simulink model "lab5_sim"  (R2024b)
settings: Solver=VariableStepAuto  StartTime=0.0  StopTime=0.3  RelTol=1e-3
values from neighbouring files (symbols this model uses):
  A = [-Ra/La, -K/La; K/J, 0;]    [Lab5.m]    (also in Lab5_recapitulare.m)
  A_d = double(expm(A_aux))    [Lab5.m]    (also in Lab5_recapitulare.m = double(expm(A * h)))
  B = [1/La, 0; 0, -1/J]    [Lab5.m]    (also in Lab5_recapitulare.m)
  B_d = double(int(expm(A * t) * B, 0, h))    [Lab5.m]    (also in Lab5_recapitulare.m)
  C = [1, 0; 0, 1]    [Lab5.m]    (also in Lab5_recapitulare.m)
  C_d = C    [Lab5.m]    (also in Lab5_recapitulare.m)
  D = [0, 0; 0, 0]    [Lab5.m]    (also in Lab5_recapitulare.m)
  D_d = D    [Lab5.m]    (also in Lab5_recapitulare.m)
  h = 0.01    [Lab5.m]    (also in Lab5_recapitulare.m)
undefined symbols (not defined in the file or in its folder): denz1, denz2, numz1, numz2
settings Model: Creator=akopo  LastModifiedBy=akopo

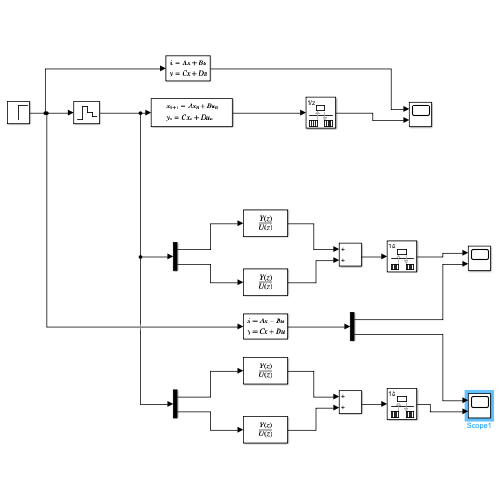
[thumbnail: Simulink's stored preview of the top-level diagram]
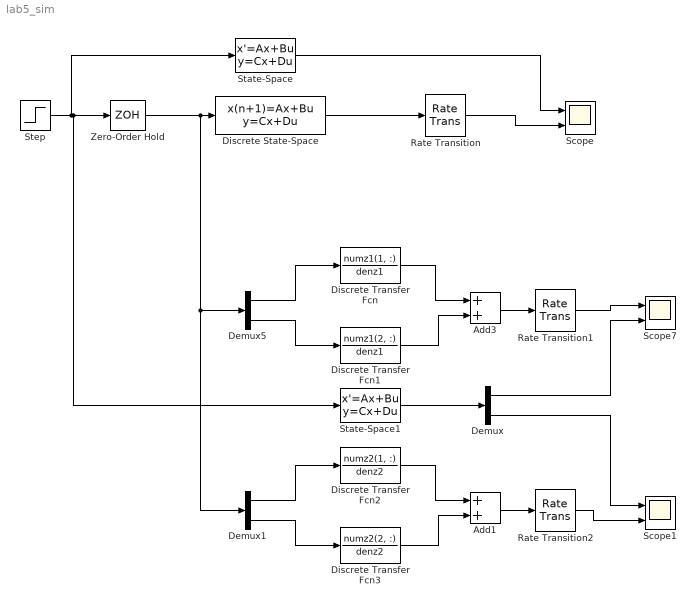
== system lab5_sim ==
  Add1 : Sum
  Add3 : Sum
  Demux : Demux  Outputs=2
  Demux1 : Demux  Outputs=2
  Demux5 : Demux  Outputs=2
  Discrete Transfer Fcn : DiscreteTransferFcn  Numerator=numz1(1, :)  Denominator=denz1
  Discrete Transfer Fcn1 : DiscreteTransferFcn  Numerator=numz1(2, :)  Denominator=denz1
  Discrete Transfer Fcn2 : DiscreteTransferFcn  Numerator=numz2(1, :)  Denominator=denz2
  Discrete Transfer Fcn3 : DiscreteTransferFcn  Numerator=numz2(2, :)  Denominator=denz2
  Discrete State-Space : DiscreteStateSpace  A=A_d  B=B_d  C=C_d  D=D_d  SampleTime=h
  Rate Transition : RateTransition
  Rate Transition1 : RateTransition
  Rate Transition2 : RateTransition
  Scope : Scope  NumInputPorts=2
  Scope1 : Scope  NumInputPorts=2
  Scope7 : Scope  NumInputPorts=2
  State-Space : StateSpace  A=A  B=B  C=C  D=D  InitialCondition=0
  State-Space1 : StateSpace  A=A  B=B  C=C  D=D  InitialCondition=0
  Step : Step  Time=0  Before=[0, 0]  After=[24; 0.04]  SampleTime=h
  Zero-Order Hold : ZeroOrderHold  SampleTime=h
  wires:
  Rate Transition/1 -> Scope/2
  Step/1 -> State-Space/1, State-Space1/1, Zero-Order Hold/1
  Discrete State-Space/1 -> Rate Transition/1
  State-Space/1 -> Scope/1
  Demux5/1 -> Discrete Transfer Fcn/1
  Demux5/2 -> Discrete Transfer Fcn1/1
  Discrete Transfer Fcn1/1 -> Add3/2
  Discrete Transfer Fcn/1 -> Add3/1
  Add3/1 -> Rate Transition1/1
  Rate Transition1/1 -> Scope7/1
  Rate Transition2/1 -> Scope1/2
  Demux1/2 -> Discrete Transfer Fcn3/1
  Add1/1 -> Rate Transition2/1
  Discrete Transfer Fcn3/1 -> Add1/2
  Demux1/1 -> Discrete Transfer Fcn2/1
  Discrete Transfer Fcn2/1 -> Add1/1
  Zero-Order Hold/1 -> Demux1/1, Demux5/1, Discrete State-Space/1
  State-Space1/1 -> Demux/1
  Demux/1 -> Scope7/2
  Demux/2 -> Scope1/1
